simulink model "EcoSIM3_P2_C2_WIP"  (R2014b)
settings: Solver=ode1  SolverMode=SingleTasking  StartTime=0.0  StopTime=4  FixedStep=0.01  RelTol=1e-3
PostLoadFcn:
  | %, if any(exist('dsrtsu_mdlpostloadfcn', 'file') == [2, 3, 6]), try dsrtsu_mdlpostloadfcn('Execute', bdroot); catch fprintf('Error in PostLoadFcn (dsrtsu_mdlpostloadfcn) for model "%s":\n %s\n', bdroot, lasterr); end, end,
InitFcn:
  | tic
  | %Startup_EcoSIM
undefined symbols (not defined in the file or in its folder): canChannel, Controls, DriveCycles, Driver, EM_EFF_MAP, EM_PwrLoss_MAP, EngPwr, EngSpd, EngTrq, Glbl, Overwritten_Mode, Plants, Power, sigbuilder_block, Torque, Trialmap, Veh_Dynamics
libraries: simulink x135, canmsglib x113, fl_lib x104, canlib x89, nesl_utility x56, sdl_lib x29, dspsigops x6, dspswit3 x5, dspstat3 x2, commnoisgen2 x1, dspfdesign x1
(part 8 of 21)

== system EcoSIM3_P2_C2_WIP/Supervisory Controller/Input Conditioning/Velocity Conditioning/Subsystem2 ==
  In1 : Inport
  Add : Sum  Inputs=+-
  Delay : Delay  DelayLength=50
  Gain6 : Gain  Gain=2*pi
  Memory2 : Memory
  Product2 : Product  Inputs=*/
  Product3 : Product  Inputs=*/
  Product4 : Product
  Scope8 : Scope
      settings: SaveName=ScopeData21
  Switch2 : Switch
  Ticks_per_rev : Constant  Value=48
  TimeDiff : Constant  Value=0.5
  Transfer Fcn1 : TransferFcn  Numerator=[4]  Denominator=[1 4]
  Tyre_rad_m : Constant  Value=Plants.Rear_wh.Tire.rollrad
  m/s to km/hr1 : Gain  Gain=1/1000*3600
  Speed_LND : Outport
  wires:
  Ticks_per_rev/1 -> Product3/2
  Tyre_rad_m/1 -> Gain6/1
  In1/1 -> Add/1, Delay/1
  Switch2/1 -> Transfer Fcn1/1, Memory2/1
  Product4/1 -> Speed_LND/1, m/s to km/hr1/1  "Left_NonDriven_mps_delay"
  Delay/1 -> Add/2
  Product2/1 -> Switch2/2, Switch2/1
  TimeDiff/1 -> Product2/2
  Memory2/1 -> Switch2/3
  Transfer Fcn1/1 -> Product3/1
  m/s to km/hr1/1 -> Scope8/1  "Left_NonDriven_kph"
  Gain6/1 -> Product4/2
  Product3/1 -> Product4/1
  Add/1 -> Product2/1

== system EcoSIM3_P2_C2_WIP/Supervisory Controller/Input Conditioning/Velocity Conditioning/Subsystem3 ==
  In1 : Inport
  Add : Sum  Inputs=+-
  Delay : Delay  DelayLength=50
  Gain6 : Gain  Gain=2*pi
  Memory2 : Memory
  Product2 : Product  Inputs=*/
  Product3 : Product  Inputs=*/
  Product4 : Product
  Scope8 : Scope
      settings: SaveName=ScopeData21
  Switch2 : Switch
  Ticks_per_rev : Constant  Value=48
  TimeDiff : Constant  Value=0.5
  Transfer Fcn1 : TransferFcn  Numerator=[4]  Denominator=[1 4]
  Tyre_rad_m : Constant  Value=Plants.Rear_wh.Tire.rollrad
  m/s to km/hr1 : Gain  Gain=1/1000*3600
  Speed_RND : Outport
  wires:
  Add/1 -> Product2/1
  Product3/1 -> Product4/1
  Gain6/1 -> Product4/2
  m/s to km/hr1/1 -> Scope8/1  "Right_NonDriven_kph"
  Transfer Fcn1/1 -> Product3/1
  Memory2/1 -> Switch2/3
  TimeDiff/1 -> Product2/2
  Product2/1 -> Switch2/1, Switch2/2
  Delay/1 -> Add/2
  Product4/1 -> m/s to km/hr1/1, Speed_RND/1  "Right_NonDriven_mps_delay"
  Switch2/1 -> Memory2/1, Transfer Fcn1/1
  In1/1 -> Delay/1, Add/1
  Tyre_rad_m/1 -> Gain6/1
  Ticks_per_rev/1 -> Product3/2

== system EcoSIM3_P2_C2_WIP/Supervisory Controller/Mode Operation/Accessory/BAS_Signals ==
  Bus Creator4 : BusCreator  Inputs=3
  Constant1 : Constant  Value=0
  Constant4 : Constant  Value=0
  Constant5 : Constant  Value=0
  Out1 : Outport
  wires:
  Constant5/1 -> Bus Creator4/3  "BAS_Mode_Request"
  Constant4/1 -> Bus Creator4/1  "BAS_Torque_Request_Nm"
  Bus Creator4/1 -> Out1/1  "BAS_SoftECU_Receive"
  Constant1/1 -> Bus Creator4/2  "BAS_Speed_Request"

== system EcoSIM3_P2_C2_WIP/Supervisory Controller/Mode Operation/Accessory/BAS_Signals1 ==
  note: Code: Helps to set the current limits (Id and Iq)
      |
      | Write: Ensures to use the sent Id and Iq commands to the BAS inverter
      |
      | Mode Request: Always 1 for torque control mode (2 is speed control mode which is never used)
  BAS_Speed : Inport
  Bus Creator : BusCreator  Inputs=7
  Bus Selector : BusSelector  OutputSignals=BAS_Transmit.BAS_CAN_Out.Status_1.BAS_Speed_rad_per_s
  Code : Constant
  Constant : Constant  Value=0
  Gain : Gain  Gain=9.54929659643
  Gain1 : Gain
  Gain16 : Gain  Gain=-1
  Gain4 : Gain  Gain=-1
  IDLimit : Constant  Value=190
  IQLimit : Constant  Value=175.7
  Id Lookup : Lookup_n-D  BreakpointsForDimension1=Plants.BAS.Mdl.Plant.Torque  BreakpointsForDimension2=Plants.BAS.Mdl.Plant.Rpm  Table=Plants.BAS.Mdl.Plant.ID_lookup  InternalRulePriority=Speed  RndMeth=Simplest  InputSameDT=on
  Iq Lookup : Lookup_n-D  BreakpointsForDimension1=Plants.BAS.Mdl.Plant.Torque  BreakpointsForDimension2=Plants.BAS.Mdl.Plant.Rpm  Table=Plants.BAS.Mdl.Plant.IQ_Lookup  InternalRulePriority=Speed  RndMeth=Simplest  InputSameDT=on
  Max Torque Lookup : Lookup_n-D  NumberOfTableDimensions=1  BreakpointsForDimension1=Plants.BAS.Mdl.Plant.Rpm  Table=Plants.BAS.Mdl.Plant.Allowed_torque  InternalRulePriority=Speed  RndMeth=Simplest  InputSameDT=on
  Torque Saturation : simulink/Discontinuities/Saturation Dynamic  OutMin=[]  OutMax=[]  OutDataTypeStr=Inherit: Same as second input  OutDataType=fixdt(1, 16)  OutScaling=2^-10  DoSatur=off
  Torque_Request_Nm : Constant  Value=0
  "Write " : Constant
  Signals : Outport
  wires:
  "Write "/1 -> Bus Creator/1  "Write"
  IQLimit/1 -> Bus Creator/4  "IQ_Limit"
  Max Torque Lookup/1 -> Gain16/1, Torque Saturation/1
  Gain16/1 -> Torque Saturation/3
  Gain4/1 -> Bus Creator/3  "ID_Limit"
  Id Lookup/1 -> Bus Creator/6  "ID_Command"
  Bus Creator/1 -> Signals/1  "BAS_Infineon_Messages"
  IDLimit/1 -> Gain4/1  "ID_Limit"
  Torque Saturation/1 -> Iq Lookup/1, Id Lookup/1
  Gain1/1 -> Bus Creator/5  "ModeReq"
  Iq Lookup/1 -> Bus Creator/7  "IQ_Command"
  Gain/1 -> Iq Lookup/2, Id Lookup/2, Max Torque Lookup/1
  Code/1 -> Bus Creator/2  "Code"
  Bus Selector/1 -> Gain/1  "<BAS_Speed_rad_per_s>"
  BAS_Speed/1 -> Bus Selector/1
  Constant/1 -> Gain1/1  "BAS_Mode_Request"
  Torque_Request_Nm/1 -> Torque Saturation/2

== system EcoSIM3_P2_C2_WIP/Supervisory Controller/Mode Operation/Accessory/DC//DC Enabled ==
  Bus Creator : BusCreator  Inputs=3
  Constant : Constant
  Constant1 : Constant  Value=12.8
  Constant2 : Constant
  Out1 : Outport
  wires:
  Constant/1 -> Bus Creator/1  "LowVoltEnablRq"
  Constant1/1 -> Bus Creator/2  "LwVltStpntCmnd"
  Constant2/1 -> Bus Creator/3  "PrplsnSysAtv"
  Bus Creator/1 -> Out1/1  "DC_DC"

== system EcoSIM3_P2_C2_WIP/Supervisory Controller/Mode Operation/Accessory/ESS_Messages ==
  Bus Creator2 : BusCreator
  Constant : Constant
  Constant1 : Constant
  Constant2 : Constant
  Constant3 : Constant  Value=0
  Out1 : Outport
  wires:
  Constant/1 -> Bus Creator2/3  "hsc_bcm_leakage_ena"
  Constant2/1 -> Bus Creator2/1  "hsc_bcm_enable"
  Constant1/1 -> Bus Creator2/2  "hsc_bcm_mainc_close"
  Bus Creator2/1 -> Out1/1  "ESS_Signals_A123"
  Constant3/1 -> Bus Creator2/4  "hsc_bcm_epo"

== system EcoSIM3_P2_C2_WIP/Supervisory Controller/Mode Operation/Accessory/Engine Messages ==
  Bus Creator2 : BusCreator  Inputs=3
  Constant1 : Constant  Value=0
  Constant2 : Constant  Value=0
  Constant3 : Constant  Value=0
  Out1 : Outport
  wires:
  Constant1/1 -> Bus Creator2/1  "ICE_Torque_Request_Nm"
  Constant2/1 -> Bus Creator2/2  "Engine_On"
  Constant3/1 -> Bus Creator2/3  "Engine_Run"
  Bus Creator2/1 -> Out1/1  "ICE_Request"

== system EcoSIM3_P2_C2_WIP/Supervisory Controller/Mode Operation/Accessory/TM Messages ==
  Bus Creator3 : BusCreator  Inputs=3
  Constant1 : Constant  Value=0
  Constant3 : Constant  Value=0
  Constant6 : Constant  Value=0
  Out1 : Outport
  wires:
  Bus Creator3/1 -> Out1/1  "EM_Messages_Rhinehart"
  Constant1/1 -> Bus Creator3/1  "Inverter_Enable"
  Constant6/1 -> Bus Creator3/2  "Torque_Command"
  Constant3/1 -> Bus Creator3/3  "Rotation_Direction"

== system EcoSIM3_P2_C2_WIP/Supervisory Controller/Mode Operation/Accessory/Trans_Messages ==
  Bus Creator3 : BusCreator  Inputs=2
  Constant8 : Constant  Value=0
  Constant9 : Constant  Value=0
  Out1 : Outport
  wires:
  Constant9/1 -> Bus Creator3/2  "Gear_Request"
  Constant8/1 -> Bus Creator3/1  "Shift_Request"
  Bus Creator3/1 -> Out1/1  "Trans_Recieve"

== system EcoSIM3_P2_C2_WIP/Supervisory Controller/Mode Operation/Charging/BAS_Signals ==
  Bus Creator4 : BusCreator  Inputs=3
  Constant1 : Constant  Value=0
  Constant4 : Constant  Value=0
  Constant5 : Constant  Value=0
  Out1 : Outport
  wires:
  Constant5/1 -> Bus Creator4/3  "BAS_Mode_Request"
  Constant4/1 -> Bus Creator4/1  "BAS_Torque_Request_Nm"
  Bus Creator4/1 -> Out1/1  "BAS_SoftECU_Receive"
  Constant1/1 -> Bus Creator4/2  "BAS_Speed_Request"

== system EcoSIM3_P2_C2_WIP/Supervisory Controller/Mode Operation/Charging/BAS_Signals1 ==
  note: Code: Helps to set the current limits (Id and Iq)
      |
      | Write: Ensures to use the sent Id and Iq commands to the BAS inverter
      |
      | Mode Request: Always 1 for torque control mode (2 is speed control mode which is never used)
  BAS_Speed : Inport
  Bus Creator : BusCreator  Inputs=7
  Bus Selector : BusSelector  OutputSignals=BAS_Transmit.BAS_CAN_Out.Status_1.BAS_Speed_rad_per_s
  Code : Constant
  Constant : Constant  Value=0
  Gain : Gain  Gain=9.54929659643
  Gain1 : Gain
  Gain16 : Gain  Gain=-1
  Gain4 : Gain  Gain=-1
  IDLimit : Constant  Value=190
  IQLimit : Constant  Value=175.7
  Id Lookup : Lookup_n-D  BreakpointsForDimension1=Plants.BAS.Mdl.Plant.Torque  BreakpointsForDimension2=Plants.BAS.Mdl.Plant.Rpm  Table=Plants.BAS.Mdl.Plant.ID_lookup  InternalRulePriority=Speed  RndMeth=Simplest  InputSameDT=on
  Iq Lookup : Lookup_n-D  BreakpointsForDimension1=Plants.BAS.Mdl.Plant.Torque  BreakpointsForDimension2=Plants.BAS.Mdl.Plant.Rpm  Table=Plants.BAS.Mdl.Plant.IQ_Lookup  InternalRulePriority=Speed  RndMeth=Simplest  InputSameDT=on
  Max Torque Lookup : Lookup_n-D  NumberOfTableDimensions=1  BreakpointsForDimension1=Plants.BAS.Mdl.Plant.Rpm  Table=Plants.BAS.Mdl.Plant.Allowed_torque  InternalRulePriority=Speed  RndMeth=Simplest  InputSameDT=on
  Torque Saturation : simulink/Discontinuities/Saturation Dynamic  OutMin=[]  OutMax=[]  OutDataTypeStr=Inherit: Same as second input  OutDataType=fixdt(1, 16)  OutScaling=2^-10  DoSatur=off
  Torque_Request_Nm : Constant  Value=0
  "Write " : Constant
  Signals : Outport
  wires:
  "Write "/1 -> Bus Creator/1  "Write"
  IQLimit/1 -> Bus Creator/4  "IQ_Limit"
  Max Torque Lookup/1 -> Gain16/1, Torque Saturation/1
  Gain16/1 -> Torque Saturation/3
  Gain4/1 -> Bus Creator/3  "ID_Limit"
  Id Lookup/1 -> Bus Creator/6  "ID_Command"
  Bus Creator/1 -> Signals/1  "BAS_Infineon_Messages"
  IDLimit/1 -> Gain4/1  "ID_Limit"
  Torque Saturation/1 -> Iq Lookup/1, Id Lookup/1
  Gain1/1 -> Bus Creator/5  "ModeReq"
  Iq Lookup/1 -> Bus Creator/7  "IQ_Command"
  Gain/1 -> Iq Lookup/2, Id Lookup/2, Max Torque Lookup/1
  Code/1 -> Bus Creator/2  "Code"
  Bus Selector/1 -> Gain/1  "<BAS_Speed_rad_per_s>"
  BAS_Speed/1 -> Bus Selector/1
  Constant/1 -> Gain1/1  "BAS_Mode_Request"
  Torque_Request_Nm/1 -> Torque Saturation/2

== system EcoSIM3_P2_C2_WIP/Supervisory Controller/Mode Operation/Charging/DC//DC Enabled ==
  Bus Creator : BusCreator  Inputs=3
  Constant : Constant
  Constant1 : Constant  Value=12.8
  Constant2 : Constant
  Out1 : Outport
  wires:
  Constant/1 -> Bus Creator/1  "LowVoltEnablRq"
  Constant1/1 -> Bus Creator/2  "LwVltStpntCmnd"
  Constant2/1 -> Bus Creator/3  "PrplsnSysAtv"
  Bus Creator/1 -> Out1/1  "DC_DC"

== system EcoSIM3_P2_C2_WIP/Supervisory Controller/Mode Operation/Charging/EM_Signals ==
  Bus Creator3 : BusCreator  Inputs=3
  Constant1 : Constant  Value=0
  Constant3 : Constant  Value=0
  Constant6 : Constant  Value=0
  Out1 : Outport
  wires:
  Bus Creator3/1 -> Out1/1  "EM_Messages_Rhinehart"
  Constant6/1 -> Bus Creator3/2  "Torque_Command"
  Constant3/1 -> Bus Creator3/3  "Rotation_Direction"
  Constant1/1 -> Bus Creator3/1  "Inverter_Enable"

== system EcoSIM3_P2_C2_WIP/Supervisory Controller/Mode Operation/Charging/ESS_Messages ==
  From CAN : Inport
  Bus Creator1 : BusCreator
  Bus Selector1 : BusSelector  OutputSignals=ESS_Transmit.ESS_CAN_Out.BCM_Status.bcm_ready,ESS_Transmit.ESS_CAN_Out.BCM_Status.bcm_cpwr_cmd,ESS_Transmit.ESS_CAN_Out.BCM_Status.bcm_cpwr_mon,ESS_Transmit.ESS_CAN_Out.BCM_Data1.bcm_veh_mon,ESS_Transmit.ESS_CAN_Out.BCM_Status.bcm_mainc_stat
  Constant4 : Constant  Value=0
  Constant5 : Constant
  ESS Handshake : Stateflow chart  TreatAsAtomicUnit=on
  Out1 : Outport
  wires:
  Bus Selector1/5 -> ESS Handshake/5(bcm_mainc_stat)  "<bcm_mainc_stat>"
  ESS Handshake/3(hsc_bcm_leakage_ena) -> Bus Creator1/3  "hsc_bcm_leakage_ena"
  ESS Handshake/1(hsc_bcm_enable) -> Bus Creator1/1  "hsc_bcm_enable"
  From CAN/1 -> Bus Selector1/1
  Bus Selector1/3 -> ESS Handshake/3(bcm_cpwr_mon)  "<bcm_cpwr_mon>"
  Bus Selector1/2 -> ESS Handshake/2(bcm_cpwr_cmd)  "<bcm_cpwr_cmd>"
  Bus Selector1/1 -> ESS Handshake/1(bcm_ready)  "<bcm_ready>"
  ESS Handshake/2(hsc_bcm_mainc_close) -> Bus Creator1/2  "hsc_bcm_mainc_close"
  Bus Creator1/1 -> Out1/1  "ESS_Signals_A123"
  Bus Selector1/4 -> ESS Handshake/4(bcm_veh_mon)  "<bcm_veh_mon>"
  Constant4/1 -> Bus Creator1/4  "hsc_bcm_epo"
  Constant5/1 -> ESS Handshake/6(Veh_Start)

== system EcoSIM3_P2_C2_WIP/Supervisory Controller/Mode Operation/Charging/Engine Messages ==
  Bus Creator2 : BusCreator  Inputs=3
  Constant1 : Constant  Value=0
  Constant2 : Constant  Value=0
  Constant3 : Constant  Value=0
  Out1 : Outport
  wires:
  Constant1/1 -> Bus Creator2/1  "ICE_Torque_Request_Nm"
  Constant2/1 -> Bus Creator2/2  "Engine_On"
  Constant3/1 -> Bus Creator2/3  "Engine_Run"
  Bus Creator2/1 -> Out1/1  "ICE_Request"

== system EcoSIM3_P2_C2_WIP/Supervisory Controller/Mode Operation/Charging/Trans_Messages ==
  Bus Creator3 : BusCreator  Inputs=2
  Constant8 : Constant  Value=0
  Constant9 : Constant  Value=0
  Out1 : Outport
  wires:
  Constant9/1 -> Bus Creator3/2  "Gear_Request"
  Constant8/1 -> Bus Creator3/1  "Shift_Request"
  Bus Creator3/1 -> Out1/1  "Trans_Recieve"

== system EcoSIM3_P2_C2_WIP/Supervisory Controller/Mode Operation/EV/BAS_Signals ==
  Bus Creator4 : BusCreator  Inputs=3
  Constant1 : Constant  Value=0
  Constant4 : Constant  Value=0
  Constant5 : Constant
  Out1 : Outport
  wires:
  Constant5/1 -> Bus Creator4/3  "BAS_Mode_Request"
  Constant4/1 -> Bus Creator4/1  "BAS_Torque_Request_Nm"
  Bus Creator4/1 -> Out1/1  "BAS_SoftECU_Receive"
  Constant1/1 -> Bus Creator4/2  "BAS_Speed_Request"

== system EcoSIM3_P2_C2_WIP/Supervisory Controller/Mode Operation/EV/BAS_Signals1 ==
  note: Code: Helps to set the current limits (Id and Iq)
      |
      | Write: Ensures to use the sent Id and Iq commands to the BAS inverter
      |
      | Mode Request: Always 1 for torque control mode (2 is speed control mode which is never used)
  BAS_Speed : Inport
  Bus Creator : BusCreator  Inputs=7
  Bus Selector : BusSelector  OutputSignals=BAS_Transmit.BAS_CAN_Out.Status_1.BAS_Speed_rad_per_s
  Code : Constant
  Constant : Constant
  Gain : Gain  Gain=9.54929659643
  Gain1 : Gain
  Gain16 : Gain  Gain=-1
  Gain4 : Gain  Gain=-1
  IDLimit : Constant  Value=190
  IQLimit : Constant  Value=175.7
  Id Lookup : Lookup_n-D  BreakpointsForDimension1=Plants.BAS.Mdl.Plant.Torque  BreakpointsForDimension2=Plants.BAS.Mdl.Plant.Rpm  Table=Plants.BAS.Mdl.Plant.ID_lookup  InternalRulePriority=Speed  RndMeth=Simplest  InputSameDT=on
  Iq Lookup : Lookup_n-D  BreakpointsForDimension1=Plants.BAS.Mdl.Plant.Torque  BreakpointsForDimension2=Plants.BAS.Mdl.Plant.Rpm  Table=Plants.BAS.Mdl.Plant.IQ_Lookup  InternalRulePriority=Speed  RndMeth=Simplest  InputSameDT=on
  Max Torque Lookup : Lookup_n-D  NumberOfTableDimensions=1  BreakpointsForDimension1=Plants.BAS.Mdl.Plant.Rpm  Table=Plants.BAS.Mdl.Plant.Allowed_torque  InternalRulePriority=Speed  RndMeth=Simplest  InputSameDT=on
  Torque Saturation : simulink/Discontinuities/Saturation Dynamic  OutMin=[]  OutMax=[]  OutDataTypeStr=Inherit: Same as second input  OutDataType=fixdt(1, 16)  OutScaling=2^-10  DoSatur=off
  Torque_Request_Nm : Constant  Value=0
  "Write " : Constant
  Signals : Outport
  wires:
  "Write "/1 -> Bus Creator/1  "Write"
  IQLimit/1 -> Bus Creator/4  "IQ_Limit"
  Max Torque Lookup/1 -> Gain16/1, Torque Saturation/1
  Gain16/1 -> Torque Saturation/3
  Gain4/1 -> Bus Creator/3  "ID_Limit"
  Id Lookup/1 -> Bus Creator/6  "ID_Command"
  Torque_Request_Nm/1 -> Torque Saturation/2
  Bus Creator/1 -> Signals/1  "BAS_Infineon_Messages"
  IDLimit/1 -> Gain4/1  "ID_Limit"
  Torque Saturation/1 -> Iq Lookup/1, Id Lookup/1
  Gain1/1 -> Bus Creator/5  "ModeReq"
  Iq Lookup/1 -> Bus Creator/7  "IQ_Command"
  Gain/1 -> Iq Lookup/2, Id Lookup/2, Max Torque Lookup/1
  Code/1 -> Bus Creator/2  "Code"
  Bus Selector/1 -> Gain/1  "<BAS_Speed_rad_per_s>"
  BAS_Speed/1 -> Bus Selector/1
  Constant/1 -> Gain1/1  "BAS_Mode_Request"

== system EcoSIM3_P2_C2_WIP/Supervisory Controller/Mode Operation/EV/DC//DC Enabled ==
  Bus Creator : BusCreator  Inputs=3
  Constant : Constant
  Constant1 : Constant  Value=12.8
  Constant2 : Constant
  Out1 : Outport
  wires:
  Constant/1 -> Bus Creator/1  "LowVoltEnablRq"
  Constant1/1 -> Bus Creator/2  "LwVltStpntCmnd"
  Constant2/1 -> Bus Creator/3  "PrplsnSysAtv"
  Bus Creator/1 -> Out1/1  "DC_DC"

== system EcoSIM3_P2_C2_WIP/Supervisory Controller/Mode Operation/EV/ESS_Messages ==
  Bus Creator2 : BusCreator
  Constant : Constant
  Constant1 : Constant
  Constant2 : Constant
  Constant3 : Constant  Value=0
  Out1 : Outport
  wires:
  Constant/1 -> Bus Creator2/3  "hsc_bcm_leakage_ena"
  Constant2/1 -> Bus Creator2/1  "hsc_bcm_enable"
  Constant1/1 -> Bus Creator2/2  "hsc_bcm_mainc_close"
  Bus Creator2/1 -> Out1/1  "ESS_Signals_A123"
  Constant3/1 -> Bus Creator2/4  "hsc_bcm_epo"

== system EcoSIM3_P2_C2_WIP/Supervisory Controller/Mode Operation/EV/Engine Messages ==
  Bus Creator2 : BusCreator  Inputs=3
  Constant1 : Constant  Value=0
  Constant2 : Constant  Value=0
  Constant3 : Constant  Value=0
  Out1 : Outport
  wires:
  Constant1/1 -> Bus Creator2/1  "ICE_Torque_Request_Nm"
  Constant2/1 -> Bus Creator2/2  "Engine_On"
  Constant3/1 -> Bus Creator2/3  "Engine_Run"
  Bus Creator2/1 -> Out1/1  "ICE_Request"

== system EcoSIM3_P2_C2_WIP/Supervisory Controller/Mode Operation/EV/Trans_Messages ==
  Bus Creator3 : BusCreator  Inputs=2
  Constant8 : Constant  Value=0
  Constant9 : Constant  Value=0
  Out1 : Outport
  wires:
  Constant9/1 -> Bus Creator3/2  "Gear_Request"
  Constant8/1 -> Bus Creator3/1  "Shift_Request"
  Bus Creator3/1 -> Out1/1  "Trans_Recieve"

== system EcoSIM3_P2_C2_WIP/Supervisory Controller/Mode Operation/Engine Only /BAS_Signals ==
  Bus Creator4 : BusCreator  Inputs=3
  Constant1 : Constant  Value=0
  Constant4 : Constant  Value=0
  Constant5 : Constant
  Out1 : Outport
  wires:
  Constant5/1 -> Bus Creator4/3  "BAS_Mode_Request"
  Constant4/1 -> Bus Creator4/1  "BAS_Torque_Request_Nm"
  Bus Creator4/1 -> Out1/1  "BAS_SoftECU_Receive"
  Constant1/1 -> Bus Creator4/2  "BAS_Speed_Request"

== system EcoSIM3_P2_C2_WIP/Supervisory Controller/Mode Operation/Engine Only /BAS_Signals1 ==
  note: Code: Helps to set the current limits (Id and Iq)
      |
      | Write: Ensures to use the sent Id and Iq commands to the BAS inverter
      |
      | Mode Request: Always 1 for torque control mode (2 is speed control mode which is never used)
  BAS_Speed : Inport
  Bus Creator : BusCreator  Inputs=7
  Bus Selector : BusSelector  OutputSignals=BAS_Transmit.BAS_CAN_Out.Status_1.BAS_Speed_rad_per_s,Alpha_percent
  Code : Constant
  Constant : Constant
  Gain : Gain  Gain=9.54929659643
  Gain1 : Gain
  Gain16 : Gain  Gain=-1
  Gain2 : Gain  Gain=60/100
  Gain4 : Gain  Gain=-1
  IDLimit : Constant  Value=190
  IQLimit : Constant  Value=175.7
  Id Lookup : Lookup_n-D  BreakpointsForDimension1=Plants.BAS.Mdl.Plant.Torque  BreakpointsForDimension2=Plants.BAS.Mdl.Plant.Rpm  Table=Plants.BAS.Mdl.Plant.ID_lookup  InternalRulePriority=Speed  RndMeth=Simplest  InputSameDT=on
  Iq Lookup : Lookup_n-D  BreakpointsForDimension1=Plants.BAS.Mdl.Plant.Torque  BreakpointsForDimension2=Plants.BAS.Mdl.Plant.Rpm  Table=Plants.BAS.Mdl.Plant.IQ_Lookup  InternalRulePriority=Speed  RndMeth=Simplest  InputSameDT=on
  Max Torque Lookup : Lookup_n-D  NumberOfTableDimensions=1  BreakpointsForDimension1=Plants.BAS.Mdl.Plant.Rpm  Table=Plants.BAS.Mdl.Plant.Allowed_torque  InternalRulePriority=Speed  RndMeth=Simplest  InputSameDT=on
  Peak Lookup : Lookup_n-D  Commented=on  NumberOfTableDimensions=1  BreakpointsForDimension1=Plants.BAS.Mdl.Plant.max_min_RPM  Table=Plants.BAS.Mdl.Plant.T_max_Peak  InternalRulePriority=Speed  RndMeth=Simplest  InputSameDT=on
  Scope1 : Scope  NumInputPorts=3
      settings: YMin=-5~-5~-5  YMax=5~5~5  SaveName=ScopeData26
  Terminator : Terminator
  Torque Saturation : simulink/Discontinuities/Saturation Dynamic  OutMin=[]  OutMax=[]  OutDataTypeStr=Inherit: Same as second input  OutDataType=fixdt(1, 16)  OutScaling=2^-10  DoSatur=off
  Torque_Request_Nm : Constant  Value=0
  "Write " : Constant
  Signals : Outport
  wires:
  "Write "/1 -> Bus Creator/1  "Write"
  IQLimit/1 -> Bus Creator/4  "IQ_Limit"
  Max Torque Lookup/1 -> Gain16/1, Torque Saturation/1
  Gain16/1 -> Torque Saturation/3
  Gain4/1 -> Bus Creator/3  "ID_Limit"
  Id Lookup/1 -> Scope1/2, Bus Creator/6  "ID_Command"
  Bus Creator/1 -> Signals/1  "BAS_Infineon_Messages"
  IDLimit/1 -> Gain4/1  "ID_Limit"
  Torque Saturation/1 -> Scope1/1, Iq Lookup/1, Id Lookup/1
  Gain1/1 -> Bus Creator/5  "ModeReq"
  Iq Lookup/1 -> Scope1/3, Bus Creator/7  "IQ_Command"
  Gain/1 -> Max Torque Lookup/1, Iq Lookup/2, Id Lookup/2
  Code/1 -> Bus Creator/2  "Code"
  Bus Selector/1 -> Gain/1  "<BAS_Speed_rad_per_s>"
  BAS_Speed/1 -> Bus Selector/1
  Constant/1 -> Gain1/1  "BAS_Mode_Request"
  Bus Selector/2 -> Gain2/1  "<Alpha_percent>"
  Torque_Request_Nm/1 -> Torque Saturation/2
  Gain2/1 -> Terminator/1

== system EcoSIM3_P2_C2_WIP/Supervisory Controller/Mode Operation/Engine Only /DC//DC Enabled ==
  Bus Creator : BusCreator  Inputs=3
  Constant : Constant
  Constant1 : Constant  Value=12.8
  Constant2 : Constant
  Out1 : Outport
  wires:
  Constant/1 -> Bus Creator/1  "LowVoltEnablRq"
  Constant1/1 -> Bus Creator/2  "LwVltStpntCmnd"
  Constant2/1 -> Bus Creator/3  "PrplsnSysAtv"
  Bus Creator/1 -> Out1/1  "DC_DC"

== system EcoSIM3_P2_C2_WIP/Supervisory Controller/Mode Operation/Engine Only /ESS_Messages ==
  Bus Creator2 : BusCreator
  Constant : Constant
  Constant1 : Constant
  Constant2 : Constant
  Constant3 : Constant  Value=0
  Out1 : Outport
  wires:
  Constant/1 -> Bus Creator2/3  "hsc_bcm_leakage_ena"
  Constant2/1 -> Bus Creator2/1  "hsc_bcm_enable"
  Constant1/1 -> Bus Creator2/2  "hsc_bcm_mainc_close"
  Bus Creator2/1 -> Out1/1  "ESS_Signals_A123"
  Constant3/1 -> Bus Creator2/4  "hsc_bcm_epo"

== system EcoSIM3_P2_C2_WIP/Supervisory Controller/Mode Operation/Engine Only /Engine Messages ==
  Bus Creator2 : BusCreator  Inputs=3
  Constant1 : Constant  Value=0
  Constant2 : Constant
  Constant3 : Constant
  Out1 : Outport
  wires:
  Constant1/1 -> Bus Creator2/1  "ICE_Torque_Request_Nm"
  Constant2/1 -> Bus Creator2/2  "Engine_On"
  Constant3/1 -> Bus Creator2/3  "Engine_Run"
  Bus Creator2/1 -> Out1/1  "ICE_Request"

== system EcoSIM3_P2_C2_WIP/Supervisory Controller/Mode Operation/Engine Only /Engine Messages1 ==
  Torque : Inport
  Bus Creator2 : BusCreator  Inputs=3
  Constant2 : Constant
  Constant3 : Constant
  Gain : Gain
  Out1 : Outport
  wires:
  Gain/1 -> Bus Creator2/1  "ICE_Torque_Request_Nm"
  Constant2/1 -> Bus Creator2/2  "Engine_On"
  Constant3/1 -> Bus Creator2/3  "Engine_Run"
  Bus Creator2/1 -> Out1/1  "ICE_Request"
  Torque/1 -> Gain/1

== system EcoSIM3_P2_C2_WIP/Supervisory Controller/Mode Operation/Engine Only /ICE Torque Request & Gear Selection  ==
  note: Toggle algorithm between 'flat' and 'nearest', check difference
  note: Changing input signal affects rate limiter in engine softecu
  note: Should this be driver torque request or engine actual torque command?
  CAN : Inport
  Bus Selector : BusSelector  OutputSignals=Vehicle_speed.Vehicle_Speed_meter_per_s,ICE_Transmit.ICE_CAN_Out.ICE_Torque.ICE_Torque_Cmd_Nm,Alpha_percent,ModeSwitch_Conditioned.Propulsion_mode
  Compare To Constant : simulink/Logic and Bit Operations/Compare To Constant  relop===  const=2  OutDataTypeStr=boolean
  Constant1 : Constant
  Constant4 : Constant
  Data Type Conversion : DataTypeConversion
  Diff_GR : Gain  Gain=Plants.Rear_Diff.Diff_ratio
  Display : Display
  Max ICE torque : Gain  Gain=max(Plants.ICE.Mdl.Plant.Max_Trq.Trq)
  Memory : Memory  InheritSampleTime=on
  Multiply : Product  Inputs=**
  Product : Product
  Switch : Switch  Criteria=u2 > Threshold  Threshold=0.5
  Terminator : Terminator
  ToKph : Gain  Gain=3.6
  Trans GR : Lookup  InputValues=Plants.Trans.Mdl.Plant.Gear_cmd  Table=Plants.Trans.Mdl.Plant.GR  LookUpMeth=Use Input Nearest
  Trial gear map : Lookup_n-D  BreakpointsForDimension1=Controls.Trans.Trialmap.Vehspdkph  BreakpointsForDimension2=Controls.Trans.Trialmap.AcPedalPosn  Table=Controls.Trans.Trialmap.Gear  InterpMethod=Flat  InternalRulePriority=Speed  RndMeth=Simplest  InputSameDT=on
  optimal gear map : Lookup_n-D  BreakpointsForDimension1=Controls.Trans.shiftmap.vehspd  BreakpointsForDimension2=Controls.Trans.shiftmap.whltrq  Table=Controls.Trans.shiftmap.gear  InterpMethod=Nearest  InternalRulePriority=Speed  RndMeth=Simplest  InputSameDT=on
  percent to fraction : Gain  Gain=.01
  ICE_Torque_Request [Nm] : Outport
  Gear_Request[-] : Outport  Port=2
  wires:
  Multiply/1 -> Diff_GR/1
  percent to fraction/1 -> Max ICE torque/1
  Bus Selector/3 -> Trial gear map/2, percent to fraction/1  "<Alpha_percent>"
  Trial gear map/1 -> Gear_Request[-]/1, Memory/1  "Gear_Request"
  Trans GR/1 -> Multiply/2
  Memory/1 -> Trans GR/1
  Product/1 -> Multiply/1, ICE_Torque_Request [Nm]/1
  Bus Selector/1 -> ToKph/1, optimal gear map/1  "<Vehicle_Speed_meter_per_s>"
  Diff_GR/1 -> optimal gear map/2
  Bus Selector/4 -> Compare To Constant/1  "<Propulsion_mode>"
  Compare To Constant/1 -> Data Type Conversion/1
  Data Type Conversion/1 -> Switch/2
  Constant4/1 -> Switch/3
  Constant1/1 -> Switch/1
  Max ICE torque/1 -> Product/1
  Switch/1 -> Product/2
  CAN/1 -> Bus Selector/1
  Bus Selector/2 -> Terminator/1  "<ICE_Torque_Cmd_Nm>"
  ToKph/1 -> Trial gear map/1, Display/1

== system EcoSIM3_P2_C2_WIP/Supervisory Controller/Mode Operation/Engine Only /Subsystem ==
  From CAN : Inport
  Supervisory : Inport  Port=2
  Bus Selector : BusSelector  OutputSignals=Driver Torque Request
  Bus Selector1 : BusSelector  OutputSignals=Clutch_Transmission_SoftECU_Transmit.Clutch_Transmission_CAN_Out.Message_1.Actual_Gear,Vehicle_speed.Vehicle_Speed_meter_per_s
  Engine Torque Calc : Subsystem
  Gain : Gain  Gain=1/(2.77)
  Gear Shift Requested 1 : Subsystem
  "ICE_Torque " : Outport
  Shift Requested : Outport  Port=2
  "Gear Requested " : Outport  Port=3
  wires:
  Engine Torque Calc/1(Eng_T_Opt) -> Gain/1, Gear Shift Requested 1/3(ICE_Torque_CMD [Nm])
  From CAN/1 -> Bus Selector1/1
  Gear Shift Requested 1/1("Shift Requested ") -> Shift Requested/1
  Gear Shift Requested 1/2("Gear Requested ") -> "Gear Requested "/1
  Bus Selector/1 -> Engine Torque Calc/3(Torque Request)  "<Driver Torque Request>"
  Supervisory/1 -> Bus Selector/1
  Bus Selector1/2 -> Gear Shift Requested 1/2(Vehicle_Speed [m/s]), Engine Torque Calc/2(Vehicle Speed)  "<Vehicle_Speed_meter_per_s>"
  Bus Selector1/1 -> Engine Torque Calc/1(Gear), Gear Shift Requested 1/1("Current Gear ")  "<Actual_Gear>"
  Gain/1 -> "ICE_Torque "/1

== system EcoSIM3_P2_C2_WIP/Supervisory Controller/Mode Operation/Engine Only /TM Messages ==
  Supervisory : Inport
  CAN : Inport  Port=2
  Bus Creator2 : BusCreator  Inputs=3
  Bus Selector : BusSelector  OutputSignals=Driver Torque Request
  Bus Selector1 : BusSelector  OutputSignals=ModeSwitch_Conditioned.Propulsion_mode,EM_Transmit.EM_CAN_Out.M165_Motor_Position_Info.Motor_Speed,Alpha_percent
  Compare To Constant : simulink/Logic and Bit Operations/Compare To Constant  relop===  const=2  OutDataTypeStr=boolean
  Constant1 : Constant  Value=0
  Constant2 : Constant
  Constant4 : Constant  Value=0
  Constant6 : Constant  Value=0
  Data Type Conversion : DataTypeConversion
  EM Max Torque1 : Lookup_n-D  NumberOfTableDimensions=1  BreakpointsForDimension1=Plants.EM.Mdl.Plant.max_min_RPM  BreakpointsForDimension2=[25,70]  Table=[Plants.EM.Mdl.Plant.T_max_Peak]  InternalRulePriority=Speed  RndMeth=Simplest  InputSameDT=on
  EM Torque Request : Stateflow chart  TreatAsAtomicUnit=on
  Gain : Gain  Gain=1/(2.77*2.77)
  Gain1 : Gain
  Saturation Dynamic : simulink/Discontinuities/Saturation Dynamic  OutMin=[]  OutMax=[]  OutDataTypeStr=Inherit: Same as second input  OutDataType=fixdt(1, 16)  OutScaling=2^-10  DoSatur=off
  Switch : Switch  Criteria=u2 > Threshold  Threshold=0.5
  Terminator : Terminator
  Out1 : Outport
  wires:
  Switch/1 -> Bus Creator2/2  "Torque_Command"
  Constant1/1 -> Bus Creator2/3  "Rotation_Direction"
  Constant2/1 -> Bus Creator2/1  "Inverter_Enable"
  Bus Selector/1 -> Gain/1  "<Driver Torque Request>"
  Bus Creator2/1 -> Out1/1  "EM_Messages_Rhinehart"
  Supervisory/1 -> Bus Selector/1
  Gain/1 -> Gain1/1, EM Torque Request/1(Driver_Request)
  Constant6/1 -> Saturation Dynamic/3
  EM Max Torque1/1 -> Saturation Dynamic/1
  CAN/1 -> Bus Selector1/1
  Bus Selector1/3 -> EM Torque Request/2(Alpha)  "<Alpha_percent>"
  Bus Selector1/2 -> EM Max Torque1/1  "<Motor_Speed>"
  EM Torque Request/1(Torque_Request) -> Saturation Dynamic/2  "Torque_Command"
  Saturation Dynamic/1 -> Terminator/1  "Torque_Command"
  Compare To Constant/1 -> Data Type Conversion/1
  Data Type Conversion/1 -> Switch/2
  Constant4/1 -> Switch/3
  Gain1/1 -> Switch/1
  Bus Selector1/1 -> Compare To Constant/1  "<Propulsion_mode>"

== system EcoSIM3_P2_C2_WIP/Supervisory Controller/Mode Operation/Engine Only /Trans Clutch Messages ==
  note: 586 rpm
  note: 700 rpm
  Gear Request : Inport
  CAN : Inport  Port=2
  AggressiveClutchRelease : Stateflow chart  Commented=on  TreatAsAtomicUnit=on
  Bus Creator6 : BusCreator  Inputs=2
  Bus Selector : BusSelector  OutputSignals=BAS_Transmit.BAS_CAN_Out.Status_1.BAS_Speed_rad_per_s,Vehicle_speed.Vehicle_Speed_meter_per_s,GM_Transmit.GMLAN_CAN_Out.PPEI_Brake_Apply_Status.BrkPdlPos
  Compare To Constant1 : simulink/Logic and Bit Operations/Compare To Constant  relop=>  const=1  OutDataTypeStr=boolean
  Compare To Constant2 : simulink/Logic and Bit Operations/Compare To Constant  relop=<=  const=2  OutDataTypeStr=boolean
  Constant : Constant  Value=0.9774*Plants.ICE.Mdl.Plant.idle_w*Plants.Belt.GR
  Constant5 : Constant  Value=Plants.ICE.Mdl.Plant.clutch_w*Plants.Belt.GR
  Data Type Conversion : DataTypeConversion  OutMin=[0]  OutMax=[1]  OutDataTypeStr=double
  Display : Display
  Display1 : Display
  Display2 : Display
  Gain : Gain  Gain=0.01
  GentleClutchRelease : Stateflow chart  TreatAsAtomicUnit=on
  IC : InitialCondition  Value=0
  Logical Operator : Logic  Operator=NOT  AllPortsSameDT=off  OutDataTypeStr=boolean
  Logical Operator1 : Logic  AllPortsSameDT=off  OutDataTypeStr=boolean
  Rate Limiter : RateLimiter  Commented=on  RisingSlewLimit=inf  SampleTimeMode=inherited
  Rate Limiter1 : RateLimiter  RisingSlewLimit=inf  SampleTimeMode=inherited
  Saturation : Saturate  UpperLimit=100  LowerLimit=0
  Scope{,1..3} (4 alike) : Scope
      Scope settings: SaveName=ScopeData39
      Scope1 settings: SaveName=ScopeData40
      Scope2 settings: SaveName=ScopeData41
      Scope3 settings: SaveName=ScopeData73
  Out1 : Outport
  wires:
  IC/1 -> GentleClutchRelease/2(Clutch_Request)  "Shift_Request"
  Rate Limiter1/1 -> Scope3/1, Display2/1, Bus Creator6/1  "Shift_Request"
  CAN/1 -> Bus Selector/1
  Bus Creator6/1 -> Out1/1  "Trans_Receive"
  Compare To Constant1/1 -> Logical Operator1/2
  Gear Request/1 -> Bus Creator6/2
  Logical Operator/1 -> Data Type Conversion/1
  Logical Operator1/1 -> Logical Operator/1
  Bus Selector/3 -> Scope2/1, Compare To Constant1/1  "<BrkPdlPos>"
  Compare To Constant2/1 -> Logical Operator1/1
  Constant/1 -> GentleClutchRelease/3(Lower_Clutch_Speed), Display/1
  Constant5/1 -> GentleClutchRelease/4(Upper_Clutch_Speed), Display1/1
  Bus Selector/1 -> GentleClutchRelease/1(BAS_Speed), Scope/1  "<BAS_Speed_rad_per_s>"
  GentleClutchRelease/1(Shift_Request) -> Saturation/1
  Bus Selector/2 -> Scope1/1, Compare To Constant2/1  "<Vehicle_Speed_meter_per_s>"
  Data Type Conversion/1 -> IC/1  "Shift_Request"
  Gain/1 -> Rate Limiter1/1
  Saturation/1 -> Gain/1  "ClutchPedalPosn"

== system EcoSIM3_P2_C2_WIP/Supervisory Controller/Mode Operation/Engine Start /BAS_Signals1 ==
  note: Code: Helps to set the current limits (Id and Iq)
      |
      | Write: Ensures to use the sent Id and Iq commands to the BAS inverter
      |
      | Mode Request: Always 1 for torque control mode (2 is speed control mode which is never used)
  BAS_Speed : Inport
  1-D Lookup Table : Lookup_n-D  Commented=on  NumberOfTableDimensions=1  BreakpointsForDimension1=[0 1000 2000 2400 2500]  Table="[11.11 11.11 8 5.5  0]"  InternalRulePriority=Speed  RndMeth=Simplest  InputSameDT=on
  Bus Creator : BusCreator  Inputs=7
  Bus Selector : BusSelector  OutputSignals=BAS_Transmit.BAS_CAN_Out.Status_1.BAS_Speed_rad_per_s
  Code : Constant
  Compare To Constant : simulink/Logic and Bit Operations/Compare To Constant  Commented=on  relop=>=  const=2500  OutDataTypeStr=boolean
  Compare To Constant1 : simulink/Logic and Bit Operations/Compare To Constant  relop=>=  const=Plants.ICE.Mdl.Plant.clutch_w*Plants.Belt.GR-5  OutDataTypeStr=boolean
  Constant1 : Constant  Commented=on  Value=11.1
  Constant2 : Constant  Commented=on  Value=0
  Constant3 : Constant  Value=0
  Data Type Conversion : DataTypeConversion
  Desired_Speed : Constant  Value=Plants.ICE.Mdl.Plant.clutch_w*Plants.Belt.GR
  Display : Display
  Gain : Gain  Gain=9.54929659643
  Gain1 : Gain
  Gain16 : Gain  Gain=-1
  Gain4 : Gain  Gain=-1
  IDLimit : Constant  Value=190
  IQLimit : Constant  Value=175.7
  Id Lookup : Lookup_n-D  BreakpointsForDimension1=Plants.BAS.Mdl.Plant.Torque  BreakpointsForDimension2=Plants.BAS.Mdl.Plant.Rpm  Table=Plants.BAS.Mdl.Plant.ID_lookup  InternalRulePriority=Speed  RndMeth=Simplest  InputSameDT=on
  Iq Lookup : Lookup_n-D  BreakpointsForDimension1=Plants.BAS.Mdl.Plant.Torque  BreakpointsForDimension2=Plants.BAS.Mdl.Plant.Rpm  Table=Plants.BAS.Mdl.Plant.IQ_Lookup  InternalRulePriority=Speed  RndMeth=Simplest  InputSameDT=on
  Logical Operator : Logic  Operator=NOT  AllPortsSameDT=off  OutDataTypeStr=boolean
  Max Torque Lookup : Lookup_n-D  NumberOfTableDimensions=1  BreakpointsForDimension1=Plants.BAS.Mdl.Plant.Rpm  Table=Plants.BAS.Mdl.Plant.Allowed_torque  InternalRulePriority=Speed  RndMeth=Simplest  InputSameDT=on
  Original Lookup Table : Lookup_n-D  Commented=on  NumberOfTableDimensions=1  BreakpointsForDimension1=[0 2699 2700 3000 3239 3240]  Table=[11.11 11.11 8 5.5 5.5 0]  InternalRulePriority=Speed  RndMeth=Simplest  InputSameDT=on
  Sample and Hold : dspsigops/Sample and Hold  Commented=on  trig=Rising edge  initCond=0  latchinput=off
  Saturation : Saturate  UpperLimit=60  LowerLimit=0
  Scope : Scope  NumInputPorts=2
      settings: YMin=-5~-5  YMax=5~5  SaveName=ScopeData17
  Scope1 : Scope  NumInputPorts=3
      settings: YMin=-5~-5~-5  YMax=5~5~5  SaveName=ScopeData25
  Subsystem : Subsystem
  Switch : Switch  Commented=on  Criteria=u2 > Threshold  Threshold=0.5
  Torque Saturation : simulink/Discontinuities/Saturation Dynamic  OutMin=[]  OutMax=[]  OutDataTypeStr=Inherit: Same as second input  OutDataType=fixdt(1, 16)  OutScaling=2^-10  DoSatur=off
  "Write " : Constant
  rad/sec to RPM1 : Gain  Commented=on  Gain=1.1
  Signals : Outport
  wires:
  "Write "/1 -> Bus Creator/1  "Write"
  IQLimit/1 -> Bus Creator/4  "IQ_Limit"
  Constant3/1 -> Torque Saturation/3
  Gain4/1 -> Bus Creator/3  "ID_Limit"
  Id Lookup/1 -> Scope1/2, Bus Creator/6  "ID_Command"
  Bus Creator/1 -> Signals/1  "BAS_Infineon_Messages"
  IDLimit/1 -> Gain4/1  "ID_Limit"
  Gain1/1 -> Bus Creator/5  "ModeReq"
  Iq Lookup/1 -> Scope1/3, Bus Creator/7  "IQ_Command"
  Gain/1 -> Compare To Constant1/1, Iq Lookup/2, Id Lookup/2, Max Torque Lookup/1
  Code/1 -> Bus Creator/2  "Code"
  Bus Selector/1 -> Scope/2, Subsystem/2(BAS_Speed [rad/s]), Gain/1  "<BAS_Speed_rad_per_s>"
  BAS_Speed/1 -> Bus Selector/1
  Data Type Conversion/1 -> Gain1/1  "BAS_Mode_Request"
  Switch/1 -> rad/sec to RPM1/1  "BAS_Torque_Request_Nm"
  rad/sec to RPM1/1 -> ?  "BAS_Torque_Request_Nm"
  Compare To Constant/1 -> Sample and Hold/1, Sample and Hold/Trigger
  Sample and Hold/1 -> Switch/2  "BAS_Torque_Request_Nm"
  Constant1/1 -> Switch/3
  Constant2/1 -> Switch/1
  Subsystem/1(BAS_Torque_Request) -> Torque Saturation/2
  Compare To Constant1/1 -> Logical Operator/1
  Logical Operator/1 -> Data Type Conversion/1  "BAS_Mode_Request"
  Max Torque Lookup/1 -> Saturation/1, Gain16/1
  Saturation/1 -> Torque Saturation/1
  Desired_Speed/1 -> Display/1, Scope/1, Subsystem/1(BAS_Desired_Speed [rad/s])
  Torque Saturation/1 -> Scope1/1, Iq Lookup/1, Id Lookup/1

== system EcoSIM3_P2_C2_WIP/Supervisory Controller/Mode Operation/Engine Start /DC//DC Enabled ==
  Bus Creator : BusCreator  Inputs=3
  Constant : Constant
  Constant1 : Constant  Value=12.8
  Constant2 : Constant
  Out1 : Outport
  wires:
  Constant/1 -> Bus Creator/1  "LowVoltEnablRq"
  Constant1/1 -> Bus Creator/2  "LwVltStpntCmnd"
  Constant2/1 -> Bus Creator/3  "PrplsnSysAtv"
  Bus Creator/1 -> Out1/1  "DC_DC"

== system EcoSIM3_P2_C2_WIP/Supervisory Controller/Mode Operation/Engine Start /ESS_Messages ==
  Bus Creator2 : BusCreator
  Constant : Constant
  Constant1 : Constant
  Constant2 : Constant
  Constant3 : Constant  Value=0
  Out1 : Outport
  wires:
  Constant/1 -> Bus Creator2/3  "hsc_bcm_leakage_ena"
  Constant2/1 -> Bus Creator2/1  "hsc_bcm_enable"
  Constant1/1 -> Bus Creator2/2  "hsc_bcm_mainc_close"
  Bus Creator2/1 -> Out1/1  "ESS_Signals_A123"
  Constant3/1 -> Bus Creator2/4  "hsc_bcm_epo"

== system EcoSIM3_P2_C2_WIP/Supervisory Controller/Mode Operation/Engine Start /Engine Messages ==
  In1 : Inport
  Bus Creator3 : BusCreator  Inputs=3
  Compare To Constant1 : simulink/Logic and Bit Operations/Compare To Constant  relop=>  const=(Plants.ICE.Mdl.Plant.clutch_w*Plants.Belt.GR-5)  OutDataTypeStr=boolean
  Compare To Constant2 : simulink/Logic and Bit Operations/Compare To Constant  relop=>  const=1.5  OutDataTypeStr=boolean
  Constant : Constant  Value=(Plants.ICE.Mdl.Plant.clutch_w*Plants.Belt.GR-5)
  Constant2 : Constant
  Constant7 : Constant  Value=0
  Constant8 : Constant  Value=0
  Constant9 : Constant
  Data Type Conversion1 : DataTypeConversion  OutDataTypeStr=double
  Data Type Conversion2 : DataTypeConversion  OutDataTypeStr=double
  Display : Display
  Integrator : Integrator  ExternalReset=rising
  Switch : Switch  Criteria=u2 > Threshold  Threshold=0.5
  Out1 : Outport
  wires:
  Switch/1 -> Bus Creator3/3  "Engine_Run"
  Data Type Conversion2/1 -> Switch/2  "Engine_Run"
  Bus Creator3/1 -> Out1/1  "ICE_Request"
  Constant9/1 -> Bus Creator3/2  "Engine_On"
  Data Type Conversion1/1 -> Integrator/1, Integrator/2
  Compare To Constant2/1 -> Data Type Conversion2/1
  Integrator/1 -> Compare To Constant2/1
  Compare To Constant1/1 -> Data Type Conversion1/1
  Constant8/1 -> Bus Creator3/1  "ICE_Torque_Request_Nm"
  In1/1 -> Compare To Constant1/1
  Constant2/1 -> Switch/1
  Constant7/1 -> Switch/3
  Constant/1 -> Display/1

== system EcoSIM3_P2_C2_WIP/Supervisory Controller/Mode Operation/Engine Start /TM Messages ==
  In1 : Inport
  Bus Creator2 : BusCreator  Inputs=3
  Bus Selector : BusSelector  OutputSignals=Driver Torque Request
  Constant1 : Constant  Value=0
  Constant2 : Constant
  Gain : Gain  Gain=1/(2.77*2.77)
  Out1 : Outport
  wires:
  Gain/1 -> Bus Creator2/2  "Torque_Command"
  Constant1/1 -> Bus Creator2/3  "Rotation_Direction"
  Constant2/1 -> Bus Creator2/1  "Inverter_Enable"
  Bus Selector/1 -> Gain/1  "<Driver Torque Request>"
  Bus Creator2/1 -> Out1/1  "EM_Messages_Rhinehart"
  In1/1 -> Bus Selector/1

== system EcoSIM3_P2_C2_WIP/Supervisory Controller/Mode Operation/Engine Start /Trans Messages ==
  Bus Creator6 : BusCreator  Inputs=2
  Constant1 : Constant  Value=0
  Constant3 : Constant  Value=0
  Out1 : Outport
  wires:
  Constant3/1 -> Bus Creator6/2  "Gear_Request"
  Bus Creator6/1 -> Out1/1  "Trans_Receive"
  Constant1/1 -> Bus Creator6/1  "Shift_Request"

== system EcoSIM3_P2_C2_WIP/Supervisory Controller/Mode Operation/Limited EV/BAS_Signals ==
  Bus Creator4 : BusCreator  Inputs=3
  Constant1 : Constant  Value=0
  Constant4 : Constant  Value=0
  Constant5 : Constant
  Out1 : Outport
  wires:
  Constant5/1 -> Bus Creator4/3  "BAS_Mode_Request"
  Constant4/1 -> Bus Creator4/1  "BAS_Torque_Request_Nm"
  Bus Creator4/1 -> Out1/1  "BAS_SoftECU_Receive"
  Constant1/1 -> Bus Creator4/2  "BAS_Speed_Request"

== system EcoSIM3_P2_C2_WIP/Supervisory Controller/Mode Operation/Limited EV/BAS_Signals1 ==
  note: Code: Helps to set the current limits (Id and Iq)
      |
      | Write: Ensures to use the sent Id and Iq commands to the BAS inverter
      |
      | Mode Request: Always 1 for torque control mode (2 is speed control mode which is never used)
  BAS_Speed : Inport
  Bus Creator : BusCreator  Inputs=7
  Bus Selector : BusSelector  OutputSignals=BAS_Transmit.BAS_CAN_Out.Status_1.BAS_Speed_rad_per_s
  Code : Constant
  Constant : Constant
  Gain : Gain  Gain=9.54929659643
  Gain1 : Gain
  Gain16 : Gain  Gain=-1
  Gain4 : Gain  Gain=-1
  IDLimit : Constant  Value=190
  IQLimit : Constant  Value=175.7
  Id Lookup : Lookup_n-D  BreakpointsForDimension1=Plants.BAS.Mdl.Plant.Torque  BreakpointsForDimension2=Plants.BAS.Mdl.Plant.Rpm  Table=Plants.BAS.Mdl.Plant.ID_lookup  InternalRulePriority=Speed  RndMeth=Simplest  InputSameDT=on
  Iq Lookup : Lookup_n-D  BreakpointsForDimension1=Plants.BAS.Mdl.Plant.Torque  BreakpointsForDimension2=Plants.BAS.Mdl.Plant.Rpm  Table=Plants.BAS.Mdl.Plant.IQ_Lookup  InternalRulePriority=Speed  RndMeth=Simplest  InputSameDT=on
  Max Torque Lookup : Lookup_n-D  NumberOfTableDimensions=1  BreakpointsForDimension1=Plants.BAS.Mdl.Plant.Rpm  Table=Plants.BAS.Mdl.Plant.Allowed_torque  InternalRulePriority=Speed  RndMeth=Simplest  InputSameDT=on
  Torque Saturation : simulink/Discontinuities/Saturation Dynamic  OutMin=[]  OutMax=[]  OutDataTypeStr=Inherit: Same as second input  OutDataType=fixdt(1, 16)  OutScaling=2^-10  DoSatur=off
  Torque_Request_Nm : Constant  Value=0
  "Write " : Constant
  Signals : Outport
  wires:
  "Write "/1 -> Bus Creator/1  "Write"
  IQLimit/1 -> Bus Creator/4  "IQ_Limit"
  Max Torque Lookup/1 -> Gain16/1, Torque Saturation/1
  Gain16/1 -> Torque Saturation/3
  Gain4/1 -> Bus Creator/3  "ID_Limit"
  Id Lookup/1 -> Bus Creator/6  "ID_Command"
  Bus Creator/1 -> Signals/1  "BAS_Infineon_Messages"
  IDLimit/1 -> Gain4/1  "ID_Limit"
  Torque Saturation/1 -> Iq Lookup/1, Id Lookup/1
  Gain1/1 -> Bus Creator/5  "ModeReq"
  Iq Lookup/1 -> Bus Creator/7  "IQ_Command"
  Gain/1 -> Iq Lookup/2, Id Lookup/2, Max Torque Lookup/1
  Code/1 -> Bus Creator/2  "Code"
  Bus Selector/1 -> Gain/1  "<BAS_Speed_rad_per_s>"
  BAS_Speed/1 -> Bus Selector/1
  Constant/1 -> Gain1/1  "BAS_Mode_Request"
  Torque_Request_Nm/1 -> Torque Saturation/2

== system EcoSIM3_P2_C2_WIP/Supervisory Controller/Mode Operation/Limited EV/DC//DC Enabled ==
  Bus Creator : BusCreator  Inputs=3
  Constant : Constant
  Constant1 : Constant  Value=12.8
  Constant2 : Constant
  Out1 : Outport
  wires:
  Constant/1 -> Bus Creator/1  "LowVoltEnablRq"
  Constant1/1 -> Bus Creator/2  "LwVltStpntCmnd"
  Constant2/1 -> Bus Creator/3  "PrplsnSysAtv"
  Bus Creator/1 -> Out1/1  "DC_DC"

== system EcoSIM3_P2_C2_WIP/Supervisory Controller/Mode Operation/Limited EV/ESS_Messages ==
  Bus Creator2 : BusCreator
  Constant : Constant
  Constant1 : Constant
  Constant2 : Constant
  Constant3 : Constant  Value=0
  Out1 : Outport
  wires:
  Constant/1 -> Bus Creator2/3  "hsc_bcm_leakage_ena"
  Constant2/1 -> Bus Creator2/1  "hsc_bcm_enable"
  Constant1/1 -> Bus Creator2/2  "hsc_bcm_mainc_close"
  Bus Creator2/1 -> Out1/1  "ESS_Signals_A123"
  Constant3/1 -> Bus Creator2/4  "hsc_bcm_epo"

== system EcoSIM3_P2_C2_WIP/Supervisory Controller/Mode Operation/Limited EV/ICE_torque ==
  ICE_torque_request : Inport
  CAN : Inport  Port=2
  Bus Selector : BusSelector  OutputSignals=Vehicle_speed.Vehicle_Speed_meter_per_s,ICE_Transmit.ICE_CAN_Out.ICE_Torque.ICE_Torque_Cmd_Nm
  Engine Messages1 : Subsystem
  "ICE Torque Request & Gear Selection " : Subsystem
  Terminator : Terminator
  Trans Clutch Messages : Subsystem
  ICE_Request : Outport
  Trans_Receive : Outport  Port=2
  wires:
  "ICE Torque Request & Gear Selection "/2(Gear_Request[-]) -> Trans Clutch Messages/1(Gear Request)  "Gear_Request"
  Bus Selector/1 -> "ICE Torque Request & Gear Selection "/1(Vehicle_Speed [m/s])  "<Vehicle_Speed_meter_per_s>"
  "ICE Torque Request & Gear Selection "/1(ICE_Torque_Request [Nm]) -> Engine Messages1/1(Torque)  "ICE_Torque_Request_Nm"
  ICE_torque_request/1 -> "ICE Torque Request & Gear Selection "/2(ICE_Torque_CMD [Nm]), "ICE Torque Request & Gear Selection "/3(ICE_Torque_Request)
  Trans Clutch Messages/1(Trans_Receive) -> Trans_Receive/1
  Engine Messages1/1(ICE_Request) -> ICE_Request/1
  CAN/1 -> Bus Selector/1, Trans Clutch Messages/2(CAN)
  Bus Selector/2 -> Terminator/1  "<ICE_Torque_Cmd_Nm>"

== system EcoSIM3_P2_C2_WIP/Supervisory Controller/Mode Operation/Limited EV/Inverter Temp Selection  ==
  note: or we can use this?
  note: This is taking in all of the inverter temperatures and outputing the highest one
  In1 : Inport
  Bus Selector : BusSelector  OutputSignals=EM_CAN_Out.M160_Temperature_Set_1.Module_A,EM_CAN_Out.M160_Temperature_Set_1.Module_B,EM_CAN_Out.M160_Temperature_Set_1.Module_C,EM_CAN_Out.M160_Temperature_Set_1.Gate_Driver_Board,EM_CAN_Out.M161_Temperature_Set_2.Control_Board_Temperature
  Maximum : dspstat3/Maximum  fcn=Value and Index  reset=None  InputProcessing=Columns as channels (frame based)  indexBase=One  operateOver=Each column  Dimension=1  colComp=on  operation=maximum  roiEnable=off  roiType=Rectangles  roiPortion=Entire ROI  roiOutput=Individual statistics for each ROI  roiFlag=off  accumDataTypeStr=Inherit: Same as product output  accumLastDataTypeStr=Inherit: Same as product output  roundingMode=Floor  overflowMode=off
  MinMax : MinMax  Function=max  Inputs=5
  Relational Operator{,1..3} (4 alike) : RelationalOperator  OutDataTypeStr=boolean
  Switch{,1..3} (4 alike) : Switch  Criteria=u2 > Threshold
  Out1 : Outport
  wires:
  In1/1 -> Bus Selector/1
  Bus Selector/1 -> Switch/1, Relational Operator/1  "<Module_A>"
  Bus Selector/2 -> Switch/3, Relational Operator/2  "<Module_B>"
  Bus Selector/3 -> Relational Operator1/1, Switch1/1  "<Module_C>"
  Bus Selector/4 -> Switch1/3, Relational Operator1/2  "<Gate_Driver_Board>"
  Relational Operator/1 -> Switch/2
  Switch/1 -> Switch3/1, Relational Operator3/1
  Relational Operator1/1 -> Switch1/2
  Bus Selector/5 -> Switch2/3, Relational Operator2/2  "<Control_Board_Temperature>"
  Switch1/1 -> Switch2/1, Relational Operator2/1
  Relational Operator2/1 -> Switch2/2
  Switch2/1 -> Switch3/3, Relational Operator3/2
  Relational Operator3/1 -> Switch3/2
  Switch3/1 -> Out1/1  "Inverter_Temp"

== system EcoSIM3_P2_C2_WIP/Supervisory Controller/Mode Operation/Limited EV/Subsystem ==
  Driver_request : Inport
  ESS discharge buffer : Inport  Port=2
  Add : Sum  Inputs=-+
  Constant3 : Constant
  Constant5 : Constant
  Gain1 : Gain  Gain=1/(2.77*2.77)
  Product3 : Product
  Product4 : Product
  Switch1 : Switch  Criteria=u2 > Threshold  Threshold=0.5
  Switch3 : Switch  Criteria=u2 > Threshold  Threshold=85
  Terminator1 : Terminator
  dis_buf_limitation : Lookup_n-D  NumberOfTableDimensions=1  BreakpointsForDimension1=[20 85]  Table=[0 0.8]  ExtrapMethod=Clip  UseLastTableValue=on  InternalRulePriority=Speed  RndMeth=Simplest  InputSameDT=on
  manual_trq_split : Constant  Value=0
  trq_split_override : Constant  Value=0
  EM_trq : Outport
  ICE_trq : Outport  Port=2
  wires:
  Constant5/1 -> Add/2
  Switch1/1 -> Add/1, Product4/1  "trq_split"
  ESS discharge buffer/1 -> Switch3/2, dis_buf_limitation/1
  Product4/1 -> Gain1/1
  dis_buf_limitation/1 -> Switch3/3
  Constant3/1 -> Switch3/1
  Product3/1 -> ICE_trq/1, Terminator1/1  "ICE_trq"
  Add/1 -> Product3/2
  Driver_request/1 -> Product3/1, Product4/2
  Gain1/1 -> EM_trq/1  "EM_trq"
  Switch3/1 -> Switch1/3
  manual_trq_split/1 -> Switch1/1
  trq_split_override/1 -> Switch1/2
